simulink model "ModeloTurbinaGovernorPID"  (Simulink 7.5)
settings: Solver=ode45  StartTime=0.0  StopTime=10.0  RelTol=1e-3
undefined symbols (not defined in the file or in its folder): D1, Delta
libraries: powerlib x13
settings Model: Creator=Leandro  LastModifiedBy=Leandro
settings DebuggingCC: UnconnectedInputMsg=none  UnconnectedOutputMsg=none  UnconnectedLineMsg=none

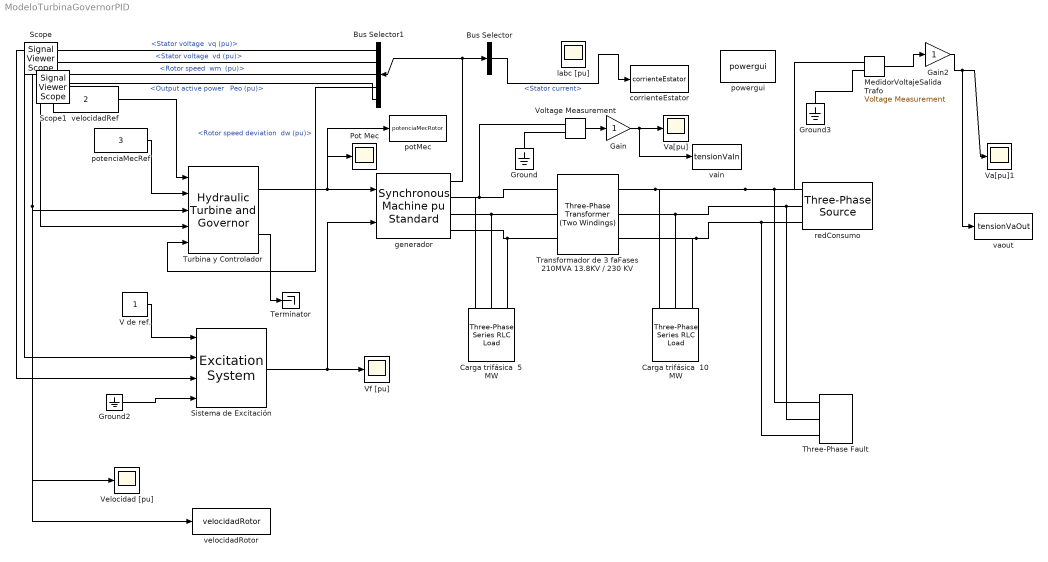
== system ModeloTurbinaGovernorPID ==
  Bus Selector : BusSelector  OutputSignals=Stator current
  Bus Selector1 : BusSelector  OutputSignals="dq0 components.Stator voltage  vq (pu),dq0 components.Stator voltage  vd (pu),Mechanical.Rotor speed  wm  (pu),Mechanical.Rotor speed deviation  dw (pu),Output active power   Peo (pu)"
  Carga trifásica  10 MW : powerlib/Elements/Three-Phase Series RLC Load  DialogController=POWERSYS.PowerSysDialog  PhysicalDomain=powersysdomain  SubClassName=unknown  LeftPortType=p1  RightPortType=p1  LConnTagsString=A|B|C  Configuration=Y (grounded)  NominalVoltage=1000  NominalFrequency=50  ActivePower=10e6  InductivePower=0  CapacitivePower=0  Measurements=None
  Carga trifásica  5 MW : powerlib/Elements/Three-Phase Series RLC Load  DialogController=POWERSYS.PowerSysDialog  PhysicalDomain=powersysdomain  SubClassName=unknown  LeftPortType=p1  RightPortType=p1  LConnTagsString=A|B|C  Configuration=Y (grounded)  NominalVoltage=1000  NominalFrequency=50  ActivePower=5e6  InductivePower=0  CapacitivePower=0  Measurements=None
  Gain : Gain  ParameterDataType=fixdt(1, 16)  ParameterScaling=2^0  OutDataType=fixdt(1, 16)  OutScaling=2^0
  Gain2 : Gain  ParameterDataType=fixdt(1, 16)  ParameterScaling=2^0  OutDataType=fixdt(1, 16)  OutScaling=2^0
  Ground : powerlib/Elements/Ground  DialogController=POWERSYS.PowerSysDialog  PhysicalDomain=powersysdomain  SubClassName=unknown  LeftPortType=p1  RightPortType=p1  LConnTagsString=a
  Ground2 : Ground
  Ground3 : powerlib/Elements/Ground  DialogController=POWERSYS.PowerSysDialog  PhysicalDomain=powersysdomain  SubClassName=unknown  LeftPortType=p1  RightPortType=p1  LConnTagsString=a
  MedidorVoltajeSalidaTrafo : powerlib/Measurements/Voltage Measurement  DialogController=POWERSYS.PowerSysDialog  SystemSampleTime=-1  PhasorSimulation=off  OutputType=Complex  PSBequivalent=0
  Pot Mec : Scope
      settings: SaveName=ScopeData2
  Sistema de Excitación : powerlib/Machines/Excitation System  DialogController=POWERSYS.PowerSysDialog  SystemSampleTime=-1  tr=20e-3  reg=[ 300, 0.001 ]  exc=[ 1, 0 ]  tgr=[ 0, 0 ]  damp=[ 0.001, 0.1 ]  sat=[ 0, 0 ]  lim=[ -11.5, 11.5, 0 ]  v0=[1,5.55628]
  Terminator : Terminator
  Three-Phase Fault : powerlib/Elements/Three-Phase Fault  DialogController=POWERSYS.PowerSysDialog  SystemSampleTime=-1  FaultA=on  FaultB=on  FaultC=on  FaultResistance=0.001  GroundFault=on  GroundResistance=0.001  External=off  SwitchStatus=[1 0]  SwitchTimes=[ 1/60 5/60]  InitialStates=[0 0 1]  SnubberResistance=1e6  SnubberCapacitance=inf  Measurements=None
  Transformador de 3 faFases 210MVA 13.8KV / 230 KV : powerlib/Elements/Three-Phase Transformer (Two Windings)  DialogController=POWERSYS.PowerSysDialog  SystemSampleTime=-1  Winding1Connection=Delta (D1)  UNITS=pu  NominalPower=[ 210e6 , 50 ]  Winding1=[ 13.8e3 , 0.002 , 0.08 ]  Winding2Connection=Yg  Winding2=[230e3 , 0.002 , 0.08 ]  SetSaturation=off  Rm=500  Lm=500  Saturation=[ 0,0 ; 0.0024,1.2 ; 1.0,1.52 ]  Hysteresis=off  DataFile='hysteresis'  SetInitialFlux=off  InitialFluxes=[ 0.8 , -0.8 , 0.7 ]  Measurements=None  MoreParameters=off  BreakLoop=off  DataType=off  TransfoNumber=1
  Turbina y Controlador : powerlib/Machines/Hydraulic Turbine and Governor  DialogController=POWERSYS.PowerSysDialog  SystemSampleTime=-1  sm="[ 10/3  0.07 ]"  gate="[  0.01  0.97518  -0.1  0.1 ]"  reg="[  0.05  1.163  0.105  0  0.01  ]"  hyd="[  0  2.67  ]"  dref=0  po=0.786957
  V de ref. : Constant  OutDataType=fixdt(1, 16)  OutScaling=2^0
  Va[pu] : Scope
      settings: YMin=-12500  YMax=12500  SaveName=ScopeData3
  Va[pu]1 : Scope
      settings: YMin=-150000  YMax=150000  SaveName=ScopeData6
  Velocidad [pu] : Scope
      settings: YMin=0.9825  YMax=1.0125
  Vf [pu] : Scope
      settings: YMin=5.5  YMax=11.5
  Voltage Measurement : powerlib/Measurements/Voltage Measurement  DialogController=POWERSYS.PowerSysDialog  SystemSampleTime=-1  PhasorSimulation=off  OutputType=Complex  PSBequivalent=0
  corrienteEstator : ToWorkspace  VariableName=corrienteEstator  SampleTime=-1  SaveFormat=Structure
  generador : powerlib/Machines/Synchronous Machine pu Standard  DialogController=POWERSYS.PowerSysDialog  SystemSampleTime=-1  PresetModel=No  MechanicalLoad=Mechanical power Pm  ShowDetailedParameters=on  RotorType=Salient-pole  NominalParameters=[210e6 13.8e3 50]  Reactances1=[ 1.81, 0.3, 0.23, 1.76, 0.65, 0.25, 0.15 ]  Reactances2="[ 1.305, 0.296, 0.252, 0.474,  0.243,  0.18 ]"  dAxisTimeConstants=Open-circuit  qAxisTimeConstants=Short-circuit  TimeConstants1="[ 4.4849  0.0681  0.1  ]"  TimeConstants2=[ 8.0, 0.03, 1.0, 0.07 ]  TimeConstants3="[  4.49  0.0681  0.0513  ]"  TimeConstants4=[ 8.0, 0.03, 0.3371, 0.0295 ]  TimeConstants5=[ 1.01, 0.053, 0.1 ]  TimeConstants6=[ 1.3201, 0.023, 1.0, 0.07 ]  TimeConstants7=[0.012 0.003 0.003]  TimeConstants8=[ 1.3201, 0.0231, 0.3371, 0.0295 ]  StatorResistance=0.003  Mechanical=[ 3.7 0 20 ]  PolePairs=20  InitialConditions=[0 -194.123 3.50983 3.50983 3.50983 170.73 50.7301 -69.2699 5.55628]  SetSaturation=off  Saturation=[0.6404,0.7127,0.8441,0.9214,0.9956,1.082,1.19,1.316,1.457;0.7,0.7698,0.8872,0.9466,0.9969,1.046,1.1,1.151,1.201]  Units=per unit standard parameters  LoadFlowParameters=[1 150000000 0 0 0]  TsPowergui=0  TsBlock=-1  IterativeModel=Forward Euler
  labc [pu] : Scope
      settings: YMin=-7  YMax=7  SaveName=ScopeData4
  potMec : ToWorkspace  VariableName=potenciaMecRotor  SampleTime=-1  SaveFormat=Structure
  potenciaMecRef : Constant  Value=3  OutDataType=fixdt(1, 16)  OutScaling=2^0
  powergui : powerlib/powergui  Priority=1  SystemSampleTime=-1  SimulationMode=Continuous  SampleTime=50e-6  frequency=60  SPID=off  DisableSnubberDevices=off  DisableRonSwitches=off  DisableVfSwitches=off  SwTol=0  Interpol=off  frequencyindice=50  echomessages=off  HookPort=off  DisplayEquations=off  FunctionMessages=off  EnableUseOfTLC=off  x0status=blocks  RestoreLinks=warning  ResistiveCurrentMeasurement=off  Ylog=off  Xlog=on  ShowGrid=off  save=off  variable=ZData  ZoomFFT=off  StartTime=0.0  cycles=1  DisplayStyle=1  FreqAxis=off  MaxFrequency=1000  frequencyindicesteady=1  display=off  methode=off
  redConsumo : powerlib/Electrical Sources/Three-Phase Source  DialogController=POWERSYS.PowerSysDialog  SystemSampleTime=-1  Voltage=230e3  PhaseAngle=0  Frequency=50  InternalConnection=Yg  SpecifyImpedance=on  Resistance=0.8929  Inductance=16.58e-3  ShortCircuitLevel=10000e6  BaseVoltage=25e3  XRratio=7
  vain : ToWorkspace  VariableName=tensionVaIn  SampleTime=-1  SaveFormat=Structure
  vaout : ToWorkspace  VariableName=tensionVaOut  SampleTime=-1  SaveFormat=Structure
  velocidadRef : Constant  Value=2  OutDataType=fixdt(1, 16)  OutScaling=2^0
  velocidadRotor : ToWorkspace  VariableName=velocidadRotor  SampleTime=-1  SaveFormat=Array
  Scope : SignalViewerScope  IOType=viewer  RefreshTime=0.035000
  Scope1 : SignalViewerScope  IOType=viewer  RefreshTime=0.035000
  wires:
  velocidadRef/1 -> Turbina y Controlador/1
  potenciaMecRef/1 -> Turbina y Controlador/2
  Turbina y Controlador/2 -> Terminator/1
  Turbina y Controlador/1 -> generador/1, Pot Mec/1, potMec/1
  V de ref./1 -> Sistema de Excitación/1
  Sistema de Excitación/1 -> generador/2, Vf [pu]/1
  generador/1 -> Bus Selector1/1, Bus Selector/1
  Bus Selector/1 -> corrienteEstator/1  "<Stator current>"
  Bus Selector1/1 -> Sistema de Excitación/3  "<Stator voltage  vq (pu)>"
  Bus Selector1/2 -> Sistema de Excitación/2  "<Stator voltage  vd (pu)>"
  Bus Selector1/3 -> Turbina y Controlador/3, velocidadRotor/1, Velocidad [pu]/1  "<Rotor speed  wm  (pu)>"
  Bus Selector1/4 -> Turbina y Controlador/5  "<Rotor speed deviation  dw (pu)>"
  Bus Selector1/5 -> Turbina y Controlador/4  "<Output active power   Peo (pu)>"
  Gain/1 -> Va[pu]/1, vain/1
  Voltage Measurement/1 -> Gain/1
  Ground2/1 -> Sistema de Excitación/4
  Gain2/1 -> Va[pu]1/1, vaout/1
  MedidorVoltajeSalidaTrafo/1 -> Gain2/1
  connections:
  generador/RConn1 -- Transformador de 3 faFases 210MVA 13.8KV / 230 KV/LConn1 -- Carga trifásica  5 MW/LConn1 -- Voltage Measurement/LConn1
  generador/RConn2 -- Transformador de 3 faFases 210MVA 13.8KV / 230 KV/LConn2 -- Carga trifásica  5 MW/LConn2
  generador/RConn3 -- Transformador de 3 faFases 210MVA 13.8KV / 230 KV/LConn3 -- Carga trifásica  5 MW/LConn3
  Voltage Measurement/LConn2 -- Ground/LConn1
  redConsumo/RConn1 -- MedidorVoltajeSalidaTrafo/LConn1 -- Transformador de 3 faFases 210MVA 13.8KV / 230 KV/RConn1 -- Carga trifásica  10 MW/LConn1 -- Three-Phase Fault/LConn1
  Transformador de 3 faFases 210MVA 13.8KV / 230 KV/RConn2 -- Carga trifásica  10 MW/LConn2 -- redConsumo/RConn2 -- Three-Phase Fault/LConn2
  Transformador de 3 faFases 210MVA 13.8KV / 230 KV/RConn3 -- Carga trifásica  10 MW/LConn3 -- redConsumo/RConn3 -- Three-Phase Fault/LConn3
  MedidorVoltajeSalidaTrafo/LConn2 -- Ground3/LConn1
